simulink library "MULTIPLIERS"  (R2019a)
settings: Solver=VariableStepAuto  StartTime=0.0  StopTime=10.0  RelTol=1e-3
libraries: xbsIndex_r4 x1
settings Model: Creator=mybur  LastModifiedBy=mybur

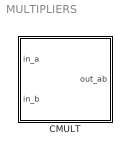
== system MULTIPLIERS ==
  CMULT : Subsystem  mask{in_a_bw=18, in_a_bp=17, in_b_bw=18, in_b_bp=17, out_ab_bw=37, out_ab_bp=34, quant_method=Round-Even, ovflw_method=Wrap, conjugate=off, is_async=off, pipeline_input=1, pipeline_product=0, pipeline_adder=1, pipeline_round=1, pipeline_output=1, use_gauss=off, use_ip=off, use_dsp=on}
      mask prompts: in_a_bw "Number of Bits 'a'"; in_a_bp "Binary Point 'a'"; in_b_bw "Number of Bits 'b'"; in_b_bp "Binary Point 'b'"; out_ab_bw "Number of Bits 'ab'"; out_ab_bp "Binary Point 'ab'"; quant_method "Quantisation"; ovflw_method "Overflow"; conjugate "Conjugate 'b'"; is_async "Is asynchronous?"; pipeline_input "Register input"; pipeline_product "Register product"; pipeline_adder "Register adder"; pipeline_round "Register round"; pipeline_output "Register output"; use_gauss "Gaussian Cmult?"; use_ip "Use IP implementation (Intel only)"; use_dsp "Use DSP?"
      mask init:
      | Simulink.Block.eval([gcb, '/cmult']);
      | 
      | cmult_subsys2bb_knit();
      mask TypeOptions quant_method: Truncate | Round-Even | Round-Inf
      mask TypeOptions ovflw_method: Wrap | Saturate
      mask TypeOptions pipeline_input: 0 | 1
      mask TypeOptions pipeline_product: 0 | 1
      mask TypeOptions pipeline_adder: 0 | 1
      mask TypeOptions pipeline_round: 0 | 1
      mask DialogControl data_tab Prompt: Data
      mask DialogControl latency_tab Prompt: Latency
      mask DialogControl implementation_tab Prompt: Implementation

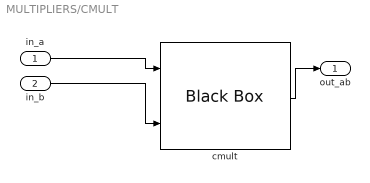
== system MULTIPLIERS/CMULT ==
  in_a : Inport
  in_b : Inport  Port=2
  cmult : xbsIndex_r4/Black Box  init_code=cmult_config  sim_method=ISE Simulator  verbose=off  block_type=blackbox2
  out_ab : Outport
  wires:
  cmult/1 -> out_ab/1
  in_a/1 -> cmult/1
  in_b/1 -> cmult/2
